simulink model "unity_img_recv"  (R2019a)
settings: Solver=VariableStepAuto  StartTime=0.0  StopTime=10.0  RelTol=1e-3
undefined symbols (not defined in the file or in its folder): f
libraries: visiongeotforms x1, instrumentlib x1
settings Model: Creator=FJJ  LastModifiedBy=FJJ

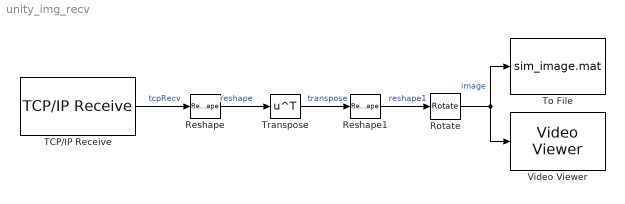
== system unity_img_recv ==
  Reshape : Reshape  OutputDimensionality=Customize  OutputDimensions=[3,307200]
  Reshape1 : Reshape  OutputDimensionality=Customize  OutputDimensions=[640,480,3]
  Rotate : visiongeotforms/Rotate  outSizeR=Expanded to fit rotated input image  src_angle=Specify via dialog  unit_angle=Degrees  angle=pi/2  maxAngle=pi  dispImage=Top-left corner  method=Table lookup  fillVal=0  interpMethod=Bilinear  roundingMode=Nearest  overflowMode=on  firstCoeffSlope=2^-10  prodOutputMode=Binary point scaling  prodOutputWordLength=32  prodOutputFracLength=10  prodOutputSlope=2^-10  accumSlope=2^-10  outputSlope=2^-10
      settings: SourceProductName=Computer Vision Toolbox
  TCP/IP Receive : instrumentlib/TCP//IP Receive  Host=127.0.0.1  Port=55555  DataSize=921600  EnableBlockingMode=on  Timeout=10  SampleTime=0.02  DataType=uint8  ByteOrder=BigEndian  ASCIIFormatting=%f,  Terminator=LF
      settings: SourceProductName=Instrument Control Toolbox
  To File : ToFile  Filename=sim_image.mat  MatrixName=panor  SaveFormat=Timeseries
  Transpose : Math  Operator=transpose  SaturateOnIntegerOverflow=on
  Video Viewer : VideoViewer  FigPos=[720.2 716.4 724.8 428.8]
  wires:
  Transpose/1 -> Reshape1/1  "transpose"
  Rotate/1 -> To File/1, Video Viewer/1  "image"
  TCP/IP Receive/1 -> Reshape/1  "tcpRecv"
  Reshape/1 -> Transpose/1  "reshape"
  Reshape1/1 -> Rotate/1  "reshape1"
